simulink model "regulator_LQG_2"  (R2021b)
settings: Solver=VariableStepAuto  StartTime=0.0  StopTime=40  RelTol=1e-3
values from neighbouring files (symbols this model uses):
  B_temp2 = [B ones(length(B),1)]    [main2.m]
  C_temp = eye(length(A))    [main2.m]
  D_temp2 = [D_temp zeros(length(D_temp),1)]    [main2.m]
  R_tilde = 1    [main2.m]
  R_tilde3 = R_tilde*100    (= 100)    [main2.m]
  x0 = [0 10]    [main2.m]
  x0_tilde = 10*x0    [main2.m]
  Z = 0    [main2.m]
undefined symbols (not defined in the file or in its folder): A, B, C, Continuous, D, k_LQ, Time
libraries: simulink x4, ctrlSharedLib x2
settings Model: Creator=PaoloA  LastModifiedBy=PaoloA

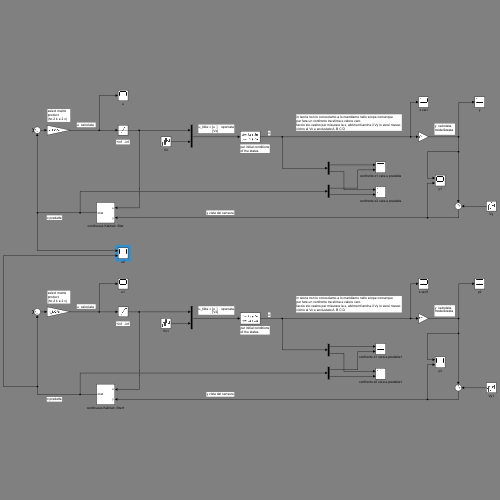
[thumbnail: Simulink's stored preview of the top-level diagram]
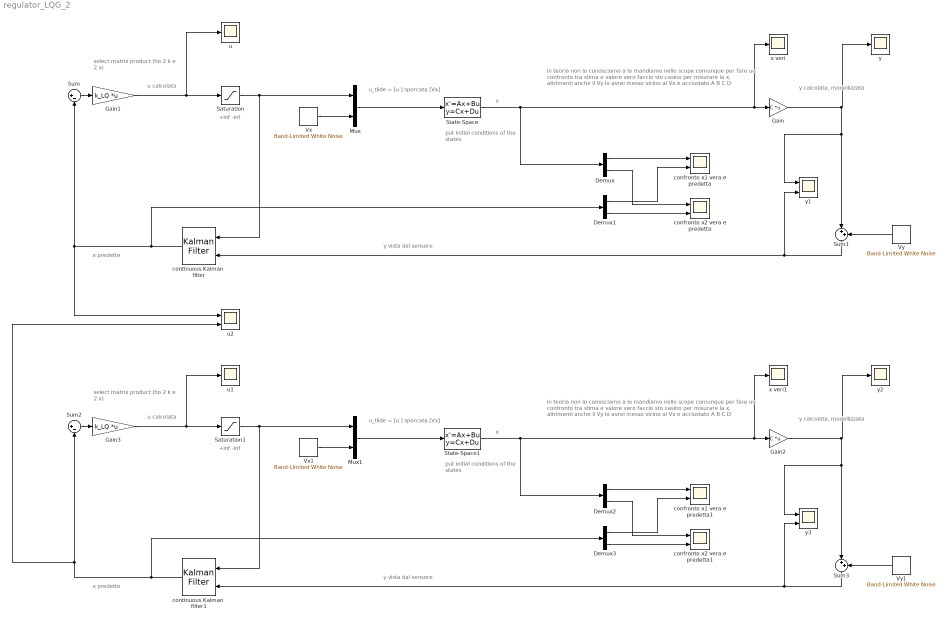
== system regulator_LQG_2 ==
  note: y vista dal sensore
  note: u_tilde = [u  ]    sporcata
      |                [Vx]
  note: x predette
  note: in teoria non lo conosciamo a lo mandiamo nello scope comunque
      | per fare un confronto tra stima e valore vero
      | faccio sto casino per misurare la x, altrimenti anche il Vy lo avrei messo
      | vicino al Vx e acciustato A  B C D
  note: select matrix
      | product
      | (ho 2 k e 2 x)
  note: y  calcolata,
      | modellizzata
  note: x
  note: u calcolata
  note: put initial conditions
      | of the states
  note: +inf -inf
  note: u calcolata
  note: x
  note: +inf -inf
  note: u_tilde = [u  ]    sporcata
      |                [Vx]
  note: x predette
  note: in teoria non lo conosciamo a lo mandiamo nello scope comunque
      | per fare un confronto tra stima e valore vero
      | faccio sto casino per misurare la x, altrimenti anche il Vy lo avrei messo
      | vicino al Vx e acciustato A  B C D
  note: select matrix
      | product
      | (ho 2 k e 2 x)
  note: y  calcolata,
      | modellizzata
  note: put initial conditions
      | of the states
  note: y vista dal sensore
  Demux{,1..3} (4 alike) : Demux  Outputs=2
  Gain : Gain  Gain=C  Multiplication=Matrix(K*u)
  Gain1 : Gain  Gain=k_LQ  Multiplication=Matrix(K*u)
  Gain2 : Gain  Gain=C  Multiplication=Matrix(K*u)
  Gain3 : Gain  Gain=k_LQ  Multiplication=Matrix(K*u)
  Mux : Mux  Inputs=2
  Mux1 : Mux  Inputs=2
  Saturation : Saturate  UpperLimit=+inf  LowerLimit=-inf
  Saturation1 : Saturate  UpperLimit=+inf  LowerLimit=-inf
  State-Space : StateSpace  A=A  B=B_temp2  C=C_temp  D=D_temp2  InitialCondition=x0
  State-Space1 : StateSpace  A=A  B=B_temp2  C=C_temp  D=D_temp2  InitialCondition=x0
  Sum : Sum  Inputs=|+-
  Sum1 : Sum  Inputs=|++
  Sum2 : Sum  Inputs=|+-
  Sum3 : Sum  Inputs=|++
  Vx : simulink/Sources/Band-Limited White Noise  Cov=power_vx  Ts=0.1  seed=[56381]
  Vx1 : simulink/Sources/Band-Limited White Noise  Cov=power_vx  Ts=0.1  seed=[56381]
  Vy : simulink/Sources/Band-Limited White Noise  Cov=power_vy  Ts=0.1  seed=[23341]
  Vy1 : simulink/Sources/Band-Limited White Noise  Cov=power_vy  Ts=0.1  seed=[23341]
  confronto x1 vera e predetta : Scope  NumInputPorts=2
  confronto x1 vera e predetta1 : Scope  NumInputPorts=2
  confronto x2 vera e predetta : Scope  NumInputPorts=2
  confronto x2 vera e predetta1 : Scope  NumInputPorts=2
  continuous Kalman  filter : ctrlSharedLib/Kalman Filter  TimeDomain=Continuous-Time  UseCurrentEstimator=on  ModelSource=Individual A, B, C, D matrices  ModelSourceVariable=ss(0.95,1,1,0,1)  A=A  B=B  C=C  D=D  NumberOfStates=1  NumberOfInputs=1  NumberOfOutputs=1  InitialEstimateSource=Dialog  X0=x0_tilde  P0=10  UseK=off  UseGH=off  NumberOfProcessNoiseInputs=1  G=1  TimeInvariantG=on  H=0  TimeInvariantH=on  Q=Q_tilde  TimeInvariantQ=on  R=R_tilde  TimeInvariantR=on  N=Z  TimeInvariantN=on  AddInputPort=on  AddEnablePort=off  OutputEstimatedY=off  OutputP=off  Ts=-1
  continuous Kalman  filter1 : ctrlSharedLib/Kalman Filter  TimeDomain=Continuous-Time  UseCurrentEstimator=on  ModelSource=Individual A, B, C, D matrices  ModelSourceVariable=ss(0.95,1,1,0,1)  A=A  B=B  C=C  D=D  NumberOfStates=1  NumberOfInputs=1  NumberOfOutputs=1  InitialEstimateSource=Dialog  X0=x0_tilde  P0=10  UseK=off  UseGH=off  NumberOfProcessNoiseInputs=1  G=1  TimeInvariantG=on  H=0  TimeInvariantH=on  Q=Q_tilde  TimeInvariantQ=on  R=R_tilde3  TimeInvariantR=on  N=Z  TimeInvariantN=on  AddInputPort=on  AddEnablePort=off  OutputEstimatedY=off  OutputP=off  Ts=-1
  u : Scope
  u1 : Scope
  u2 : Scope  NumInputPorts=2
  x veri : Scope
  x veri1 : Scope
  y : Scope
  y1 : Scope  NumInputPorts=2
  y2 : Scope
  y3 : Scope  NumInputPorts=2
  wires:
  Gain/1 -> Sum1/1, y1/1, y/1
  Sum/1 -> Gain1/1
  Gain1/1 -> u/1, Saturation/1
  Saturation/1 -> continuous Kalman  filter/1, Mux/1
  State-Space/1 -> Demux/1, Gain/1, x veri/1
  continuous Kalman  filter/1 -> Demux1/1, Sum/2, u2/1
  Sum1/1 -> y1/2, continuous Kalman  filter/2
  Vx/1 -> Mux/2
  Mux/1 -> State-Space/1
  Demux/1 -> confronto x1 vera e predetta/1
  Demux1/1 -> confronto x1 vera e predetta/2
  Demux/2 -> confronto x2 vera e predetta/1
  Demux1/2 -> confronto x2 vera e predetta/2
  Vy/1 -> Sum1/2
  Mux1/1 -> State-Space1/1
  Demux2/2 -> confronto x2 vera e predetta1/1
  Vy1/1 -> Sum3/2
  Demux3/2 -> confronto x2 vera e predetta1/2
  Demux3/1 -> confronto x1 vera e predetta1/2
  Saturation1/1 -> continuous Kalman  filter1/1, Mux1/1
  Gain3/1 -> u1/1, Saturation1/1
  Sum3/1 -> y3/2, continuous Kalman  filter1/2
  Demux2/1 -> confronto x1 vera e predetta1/1
  State-Space1/1 -> Demux2/1, Gain2/1, x veri1/1
  Gain2/1 -> Sum3/1, y3/1, y2/1
  Vx1/1 -> Mux1/2
  continuous Kalman  filter1/1 -> Demux3/1, u2/2, Sum2/2
  Sum2/1 -> Gain3/1
